simulink model "ModelSmallSize"  (R2017a)
settings: Solver=VariableStepAuto  StartTime=0.0  StopTime=5  RelTol=1e-3
values from neighbouring files (symbols this model uses):
  r = repmat(yref,N,1)    [SSmpc_ss_du_mimo.m]
  T = 0.005    [SSmpc_ss_du_mimo.m]
undefined symbols (not defined in the file or in its folder): eta, KMPC, M, Phi, u_equilibrio, w_equilibrio
undefined symbols (not defined in the file): A, B, C, CoefAtritViscMotor, CoefAtritViscRoda, ConstanteTorqueMotor, InerciaCM, InerciaMotor, InerciaRoda, l, m, redu, ResistMot, xcm, ycm
libraries: dspinverses x2
settings Model: Creator=Pichau  LastModifiedBy=arthu

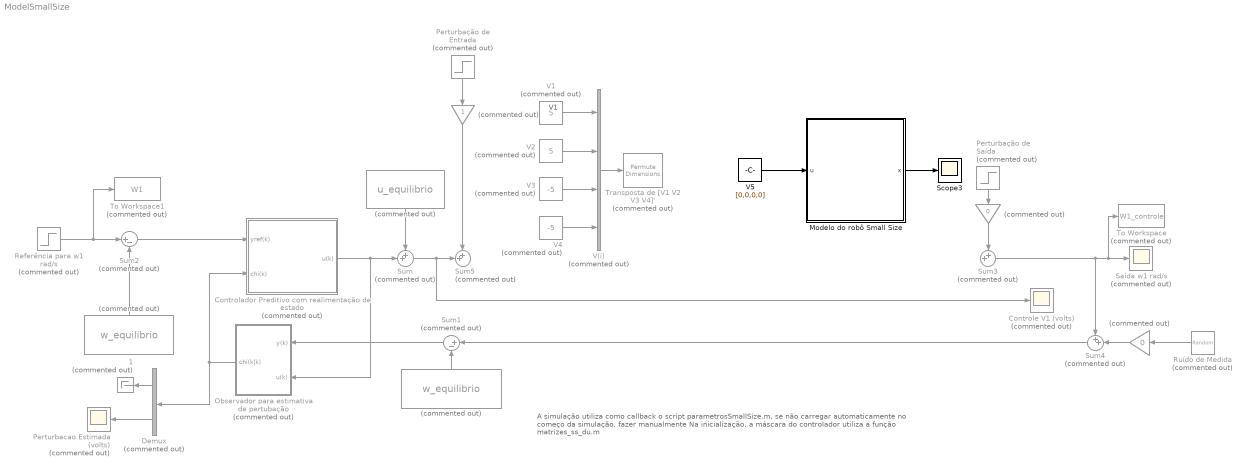
== system ModelSmallSize ==
  note: V1
  note: A simulação utiliza como callback o script parametrosSmallSize.m, se
      | não carregar automaticamente no começo da simulação, fazer manualmente
      |
      | Na inicialização, a máscara do controlador utiliza a função matrizes_ss_du.m
  " " : Constant  Commented=on  Value=w_equilibrio
  "  " : Constant  Commented=on  Value=w_equilibrio
  "   " : Constant  Commented=on  Value=u_equilibrio
  "    " : Gain  Commented=on
  "     " : Gain  Commented=on  Gain=0
  "      " : Gain  Commented=on  Gain=0
  "      1" : Terminator  Commented=on
  Controlador Preditivo com realimentação de estado : Subsystem  Commented=on  mask{rho=0.2, N=8, M=5, A=A, B=B, C=C, T=T}
      mask prompts: rho "Peso do controle (rho)"; N "Horizonte de Predição (N)"; M "Horizonte de Controle (M)"; A "Matriz A"; B "Matriz B"; C "Matriz C"; T "Periodo de amostragem"
      mask init:
      | n = size(A,1);
      | zerosn = zeros(n,1);
      | Ab = [A zerosn ; zerosn' 1];
      | Bb = [B;0];
      | Cb = [C 1];
      | [KMPC,Phi] = matrizes_ss_du(Ab,Bb,Cb,N,M,rho);
  Controle V1 (volts) : Scope  Commented=on
  Demux : Demux  Commented=on  Outputs=2
  Modelo do robô Small Size : Subsystem  mask{R=ResistMot, massa=m, raio=r, compr=l, yCM=ycm, xCM=xcm, ICM=InerciaCM, N=redu, eta=eta, Jm=InerciaMotor, Jw=InerciaRoda, k=ConstanteTorqueMotor, Bm=CoefAtritViscMotor, Bw=CoefAtritViscRoda}
      mask prompts: R "Resistência do motor"; massa "Massa do robô"; raio "Raio da roda"; compr "Distância da roda ao CM"; yCM "Y do CM"; xCM "X do CM"; ICM "Momento de inércia em relação ao CM"; N "Redução N"; eta "Eficiência do sistema de redução"; Jm "Inercia do motor Jm"; Jw "Inercia da roda Jw"; k "Constante de torque do motor K"; Bm "Coeficiente de atrito viscoso do motor Bm"; Bw "Coeficiente de atrito viscoso da roda Bw"
      mask Display: image('Glados.png');
  Observador para estimativa de pertubação : Subsystem  Commented=on  mask{A=A, B=B, C=C, T=T, poles=[0,0.02]}
      mask prompts: A "Matriz A"; B "Matriz B"; C "Matriz C"; T "Periodo de amostragem"; poles "Pólos para a dinâmica de erro de estimação"
      mask init:
      | n = size(A,1);
      | zerosn = zeros(n,1);
      | Ab = [A zerosn ; zerosn' 1];
      | Bb = [B;0];
      | Cb = [C 1];
      | L = place(Ab',Cb',poles)';
      | LL = inv(Ab)*L;
  Perturbacao Estimada (volts) : Scope  Commented=on
  Perturbação de Entrada : Step  Commented=on  Time=2  After=0.5  SampleTime=0
  Perturbação de Saída : Step  Commented=on  After=-1  SampleTime=0
  Referência para w1 rad/s : Step  Commented=on  Time=0.2  After=-0.4  SampleTime=0
  Ruído de Medida : RandomNumber  Commented=on  Variance=0.01  SampleTime=T
  Saída w1 rad/s : Scope  Commented=on
  Scope3 : Scope
  Sum{,3..5} (4 alike) : Sum  Commented=on  Inputs=++|  SaturateOnIntegerOverflow=on
  Sum1 : Sum  Commented=on  Inputs=|+-  SaturateOnIntegerOverflow=on
  Sum2 : Sum  Commented=on  Inputs=|+-  SaturateOnIntegerOverflow=on
  To Workspace : ToWorkspace  Commented=on  VariableName=W1_controle  SaveFormat=Timeseries  SampleTime=-1
      settings: Save2DSignal=2-D array (concatenate along first dimension)
  To Workspace1 : ToWorkspace  Commented=on  VariableName=W1  SaveFormat=Timeseries  SampleTime=-1
      settings: Save2DSignal=2-D array (concatenate along first dimension)
  Transposta de [V1 V2 V3 V4]' : PermuteDimensions  Commented=on  Order=[1,2]
  V(i) : Mux  Commented=on
  V1 : Constant  Commented=on  Value=5
  V2 : Constant  Commented=on  Value=5
  V3 : Constant  Commented=on  Value=-5
  V4 : Constant  Commented=on  Value=-5
  V5 : Constant  Value=[0,0,0,0]
  wires:
  V(i)/1 -> Transposta de [V1 V2 V3 V4]'/1
  V2/1 -> V(i)/2
  V3/1 -> V(i)/3
  V4/1 -> V(i)/4
  Sum3/1 -> To Workspace/1, Saída w1 rad/s/1, Sum4/1
  "      "/1 -> Sum4/2
  "   "/1 -> Sum/1
  Ruído de Medida/1 -> "      "/1
  "    "/1 -> Sum5/1
  Sum4/1 -> Sum1/1
  "     "/1 -> Sum3/1
  "  "/1 -> Sum2/2
  Perturbação de Entrada/1 -> "    "/1
  Referência para w1 rad/s/1 -> To Workspace1/1, Sum2/1
  Controlador Preditivo com realimentação de estado/1(u(k)) -> Observador para estimativa de pertubação/2(u(k)), Sum/2
  Sum/1 -> Controle V1 (volts)/1, Sum5/2
  " "/1 -> Sum1/2
  Perturbação de Saída/1 -> "     "/1
  Demux/1 -> "      1"/1
  Observador para estimativa de pertubação/1(chi(k|k)) -> Controlador Preditivo com realimentação de estado/2(chi(k)), Demux/1
  Sum2/1 -> Controlador Preditivo com realimentação de estado/1(yref(k))
  Sum1/1 -> Observador para estimativa de pertubação/1(y(k))
  Demux/2 -> Perturbacao Estimada (volts)/1
  V1/1 -> V(i)/1
  Modelo do robô Small Size/1(x) -> Scope3/1
  V5/1 -> Modelo do robô Small Size/1(u)

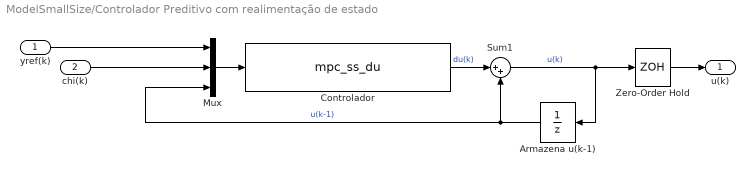
== system ModelSmallSize/Controlador Preditivo com realimentação de estado ==
  yref(k) : Inport
  chi(k) : Inport  Port=2
  Armazena u(k-1) : UnitDelay  SampleTime=T
  Controlador : S-Function  FunctionName=mpc_ss_du  Parameters=KMPC,Phi,T  SFunctionDeploymentMode=off  EnableBusSupport=off
  Mux : Mux  Inputs=3
  Sum1 : Sum  Inputs=|++  SaturateOnIntegerOverflow=on  InputSameDT=on  OutDataTypeStr=Inherit: Same as first input
  Zero-Order Hold : ZeroOrderHold  SampleTime=T
  u(k) : Outport
  wires:
  Mux/1 -> Controlador/1
  Zero-Order Hold/1 -> u(k)/1
  chi(k)/1 -> Mux/2
  yref(k)/1 -> Mux/1
  Sum1/1 -> Zero-Order Hold/1, Armazena u(k-1)/1  "u(k)"
  Armazena u(k-1)/1 -> Sum1/2, Mux/3  "u(k-1)"
  Controlador/1 -> Sum1/1  "du(k)"

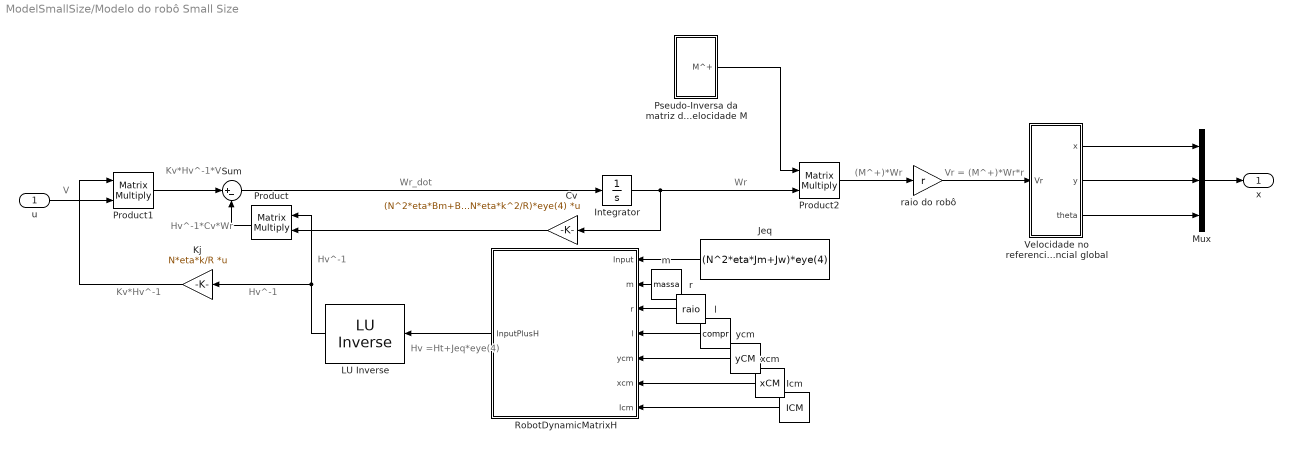
== system ModelSmallSize/Modelo do robô Small Size ==
  note: (M^+)*Wr
  note: V
  note: Kv*Hv^-1*V
  note: Hv^-1*Cv*Wr
  note: Hv =Ht+Jeq*eye(4)
  note: Wr_dot
  note: Wr
  note: Hv^-1
  note: Kv*Hv^-1
  note: Hv^-1
  note: Vr = (M^+)*Wr*r
  u : Inport
  " LU Inverse" : dspinverses/ LU Inverse
      settings: SourceProductName=DSP System Toolbox
  Cv : Gain  Gain=(N^2*eta*Bm+Bw+N*eta*k^2/R)*eye(4)  Multiplication=Matrix(K*u)
  Icm : Constant  Value=ICM
  Integrator : Integrator
  Jeq : Constant  Value=(N^2*eta*Jm+Jw)*eye(4)
  Kj : Gain  Gain=N*eta*k/R  Multiplication=Matrix(K*u)
  Mux : Mux  Inputs=3
  Product : Product  Multiplication=Matrix(*)
  Product1 : Product  Multiplication=Matrix(*)
  Product2 : Product  Multiplication=Matrix(*)
  Pseudo-Inversa da matriz de Mapeamento de velocidade M : Subsystem
  RobotDynamicMatrixH : MATLAB Function  TreatAsAtomicUnit=on
  Sum : Sum  Inputs=|+-
  Velocidade no referencial do robo para posição no referencial global : Subsystem
  l : Constant  Value=compr
  "m " : Constant  Value=massa
  r : Constant  Value=raio
  raio do robô : Gain  Gain=r
  xcm : Constant  Value=xCM
  ycm : Constant  Value=yCM
  x : Outport
  wires:
  ycm/1 -> RobotDynamicMatrixH/5(ycm)
  r/1 -> RobotDynamicMatrixH/3(r)
  xcm/1 -> RobotDynamicMatrixH/6(xcm)
  Sum/1 -> Integrator/1
  l/1 -> RobotDynamicMatrixH/4(l)
  Jeq/1 -> RobotDynamicMatrixH/1(Input)
  Icm/1 -> RobotDynamicMatrixH/7(Icm)
  "m "/1 -> RobotDynamicMatrixH/2(m)
  RobotDynamicMatrixH/1(InputPlusH) -> " LU Inverse"/1
  Product/1 -> Sum/2
  " LU Inverse"/1 -> Kj/1, Product/1
  Integrator/1 -> Product2/2, Cv/1
  Cv/1 -> Product/2
  Kj/1 -> Product1/1
  Product1/1 -> Sum/1
  u/1 -> Product1/2
  Product2/1 -> raio do robô/1
  Pseudo-Inversa da matriz de Mapeamento de velocidade M/1(M^+) -> Product2/1
  raio do robô/1 -> Velocidade no referencial do robo para posição no referencial global/1(Vr)
  Mux/1 -> x/1
  Velocidade no referencial do robo para posição no referencial global/1(x) -> Mux/1
  Velocidade no referencial do robo para posição no referencial global/2(y) -> Mux/2
  Velocidade no referencial do robo para posição no referencial global/3(theta) -> Mux/3

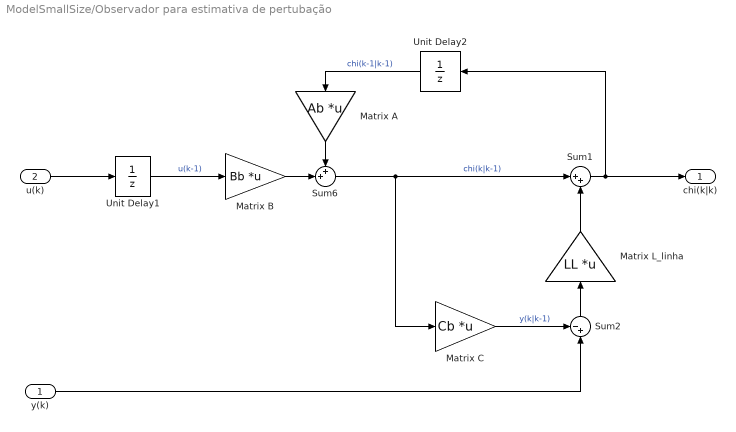
== system ModelSmallSize/Observador para estimativa de pertubação ==
  y(k) : Inport
  u(k) : Inport  Port=2
  Matrix L_linha : Gain  Gain=LL  Multiplication=Matrix(K*u)  SaturateOnIntegerOverflow=on  OutDataTypeStr=Inherit: Same as input  ParamDataTypeStr=Inherit: Same as input
  Matrix A : Gain  Gain=Ab  Multiplication=Matrix(K*u)  SaturateOnIntegerOverflow=on  OutDataTypeStr=Inherit: Same as input  ParamDataTypeStr=Inherit: Same as input
  Matrix B : Gain  Gain=Bb  Multiplication=Matrix(K*u)  SaturateOnIntegerOverflow=on  OutDataTypeStr=Inherit: Same as input  ParamDataTypeStr=Inherit: Same as input
  Matrix C : Gain  Gain=Cb  Multiplication=Matrix(K*u)  SaturateOnIntegerOverflow=on  OutDataTypeStr=Inherit: Same as input  ParamDataTypeStr=Inherit: Same as input
  Sum1 : Sum  Inputs=|++  SaturateOnIntegerOverflow=on
  Sum2 : Sum  Inputs=-+|  SaturateOnIntegerOverflow=on
  Sum6 : Sum  Inputs=++|  SaturateOnIntegerOverflow=on
  Unit Delay1 : UnitDelay  SampleTime=T
  Unit Delay2 : UnitDelay  SampleTime=T
  chi(k|k) : Outport
  wires:
  u(k)/1 -> Unit Delay1/1
  Unit Delay1/1 -> Matrix B/1  "u(k-1)"
  Matrix B/1 -> Sum6/2
  Sum6/1 -> Sum1/1, Matrix C/1  "chi(k|k-1)"
  Sum1/1 -> Unit Delay2/1, chi(k|k)/1
  Matrix A/1 -> Sum6/1
  Unit Delay2/1 -> Matrix A/1  "chi(k-1|k-1)"
  Matrix L_linha/1 -> Sum1/2
  Sum2/1 -> Matrix L_linha/1
  Matrix C/1 -> Sum2/1  "y(k|k-1)"
  y(k)/1 -> Sum2/2

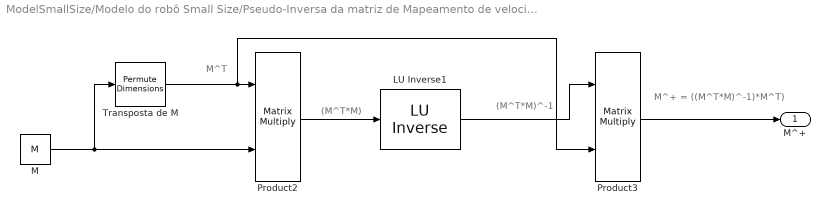
== system ModelSmallSize/Modelo do robô Small Size/Pseudo-Inversa da matriz de Mapeamento de velocidade M ==
  note: (M^T*M)
  note: M^T
  note: (M^T*M)^-1
  note: M^+ = ((M^T*M)^-1)*M^T)
  " LU Inverse1" : dspinverses/ LU Inverse
      settings: SourceProductName=DSP System Toolbox
  M : Constant  Value=M
  Product2 : Product  Multiplication=Matrix(*)
  Product3 : Product  Multiplication=Matrix(*)
  Transposta de M : PermuteDimensions
  M^+ : Outport
  wires:
  M/1 -> Product2/2, Transposta de M/1
  Product2/1 -> " LU Inverse1"/1
  Product3/1 -> M^+/1
  Transposta de M/1 -> Product3/2, Product2/1
  " LU Inverse1"/1 -> Product3/1

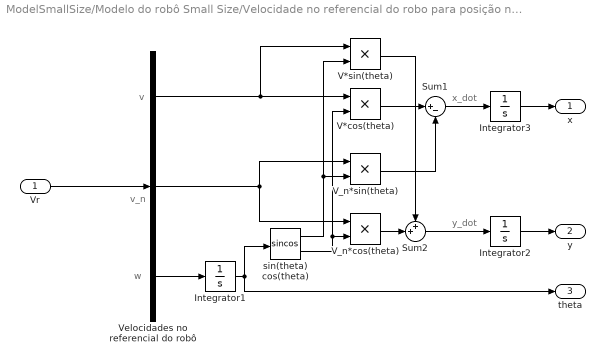
== system ModelSmallSize/Modelo do robô Small Size/Velocidade no referencial do robo para posição no referencial global ==
  note: y_dot
  note: x_dot
  note: v
  note: v_n
  note: w
  Vr : Inport
  " V_n*cos(theta)" : Product
  Integrator1 : Integrator
  Integrator2 : Integrator
  Integrator3 : Integrator
  Sum1 : Sum  Inputs=|+-
  Sum2 : Sum  Inputs=++|
  V*cos(theta) : Product
  V*sin(theta) : Product
  V_n*sin(theta) : Product
  Velocidades no referencial do robô : Demux  Outputs=3
  sin(theta) cos(theta) : Trigonometry  Operator=sincos
  x : Outport
  y : Outport  Port=2
  theta : Outport  Port=3
  wires:
  Integrator2/1 -> y/1
  V*sin(theta)/1 -> Sum2/1
  Sum2/1 -> Integrator2/1
  Integrator3/1 -> x/1
  V_n*sin(theta)/1 -> Sum1/2
  sin(theta) cos(theta)/1 -> V*sin(theta)/2, V_n*sin(theta)/2
  sin(theta) cos(theta)/2 -> V*cos(theta)/2, " V_n*cos(theta)"/2
  Velocidades no referencial do robô/2 -> " V_n*cos(theta)"/1, V_n*sin(theta)/1
  V*cos(theta)/1 -> Sum1/1
  Velocidades no referencial do robô/3 -> Integrator1/1
  Integrator1/1 -> theta/1, sin(theta) cos(theta)/1
  Vr/1 -> Velocidades no referencial do robô/1
  Velocidades no referencial do robô/1 -> V*sin(theta)/1, V*cos(theta)/1
  Sum1/1 -> Integrator3/1
  " V_n*cos(theta)"/1 -> Sum2/2

== matlab function ModelSmallSize/Modelo do robô Small Size/RobotDynamicMatrixH ==
  data: Input input; InputPlusH output; m input; r input; l input; ycm input; xcm input; Icm input
function InputPlusH = RobotDynamicMatrixH(Input,m,r,l,ycm,xcm,Icm)
%#codegen

%    This function was generated by the Symbolic Math Toolbox version 7.2.
%    07-May-2019 23:41:05

t2 = sqrt(2.0);
t3 = 1.0./l.^2;
t4 = r.^2;
t5 = xcm.^2;
t6 = m.*t5;
t7 = ycm.^2;
t8 = m.*t7;
t9 = l.*m.*t2.*ycm.*2.0;
t10 = l.^2;
t11 = m.*t10.*4.0;
t12 = l.*m.*t2.*xcm.*2.0;
t13 = Icm+t6+t8+t9;
t14 = t3.*t4.*t13.*(1.0./1.6e1);
t15 = Icm+t6+t8-t11;
t16 = t3.*t4.*t15.*(1.0./1.6e1);
t17 = Icm+t6+t8-t12;
t18 = t3.*t4.*t17.*(1.0./1.6e1);
t19 = Icm+t6+t8+t12;
t20 = t3.*t4.*t19.*(1.0./1.6e1);
t21 = Icm+t6+t8-t9;
t22 = t3.*t4.*t21.*(1.0./1.6e1);
InputPlusH = reshape([t3.*t4.*(Icm+t6+t8+t9+t11+t12).*(1.0./1.6e1),t14,t16,t20,t14,t3.*t4.*(Icm+t6+t8+t9+t11-t12).*(1.0./1.6e1),t18,t16,t16,t18,t3.*t4.*(Icm+t6+t8-t9+t11-t12).*(1.0./1.6e1),t22,t20,t16,t22,t3.*t4.*(Icm+t6+t8-t9+t11+t12).*(1.0./1.6e1)],[4,4]);
InputPlusH = (InputPlusH + Input);
